simulink model "Low_pass"  (R2018a)
settings: Solver=VariableStepAuto  StartTime=0.0  StopTime=1  RelTol=1e-3
libraries: dsparch4 x1
settings Model: Creator=AlexZ  LastModifiedBy=AlexZ
settings HardwareCC: TargetBitPerPointer=64  TargetBitPerSizeT=64  TargetBitPerPtrDiffT=64  TargetLongLongMode=on  TargetIntDivRoundTo=Zero  TargetEndianess=LittleEndian  TargetWordSize=64  TargetHWDeviceType=Custom Processor->MATLAB Host Computer  ProdEqTarget=off

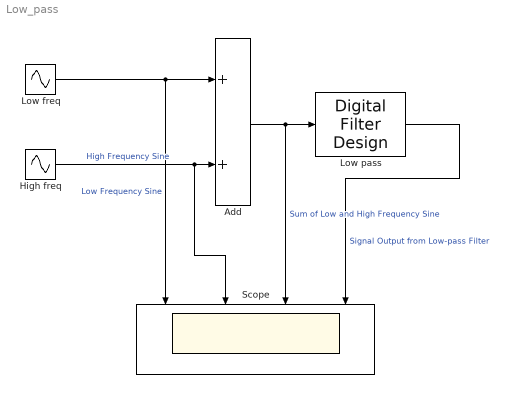
== system Low_pass ==
  Add : Sum
  "High freq " : Sin  Frequency=2*pi*50  SampleTime=0.0001
  "Low freq " : Sin  Frequency=2*pi*10  SampleTime=0.0001
  "Low pass " : dsparch4/Digital Filter Design  mwdsp_browser_bugfix_var=off
  Scope : Scope  NumInputPorts=4
  wires:
  "High freq "/1 -> Scope/2, Add/2  "High Frequency Sine"
  "Low freq "/1 -> Add/1, Scope/1  "Low Frequency Sine"
  Add/1 -> "Low pass "/1, Scope/3  "Sum of Low and High Frequency Sine"
  "Low pass "/1 -> Scope/4  "Signal Output from Low-pass Filter"
